simulink model "etc_demo_mix"  (R2017a)
settings: Solver=VariableStepAuto  StartTime=0.0  StopTime=1  RelTol=1e-3
values from neighbouring files (symbols this model uses):
  B = 0.0088    [sim_demo_set_para.m]
  den_p0 = R*Ks    (= 0.1305)    [sim_demo_set_para.m]
  den_p1 = L*Ks + R*B + Km*Kb    (= 0.1600195)    [sim_demo_set_para.m]
  den_p2 = L*B + R*J    (= 0.0031632)    [sim_demo_set_para.m]
  den_p3 = J*L    (= 3.15e-06)    [sim_demo_set_para.m]
  J = 0.0021    [sim_demo_set_para.m]
  K = 0.383    [sim_demo_set_para.m]
  Ks = 0.087    [sim_demo_set_para.m]
  L = 1.5e-3    (= 0.0015)    [sim_demo_set_para.m]
  num_i0 = Ks    (= 0.087)    [sim_demo_set_para.m]
  num_i1 = B    (= 0.0088)    [sim_demo_set_para.m]
  num_i2 = J    (= 0.0021)    [sim_demo_set_para.m]
  num_p0 = Km    (= 0.383)    [sim_demo_set_para.m]
  R = 1.5    [sim_demo_set_para.m]
  Tpl = 0.396    [sim_demo_set_para.m]
libraries: fl_lib x13, nesl_utility x6, simulink x1
settings Model: Creator=xiaopan-local  LastModifiedBy=xiaopan

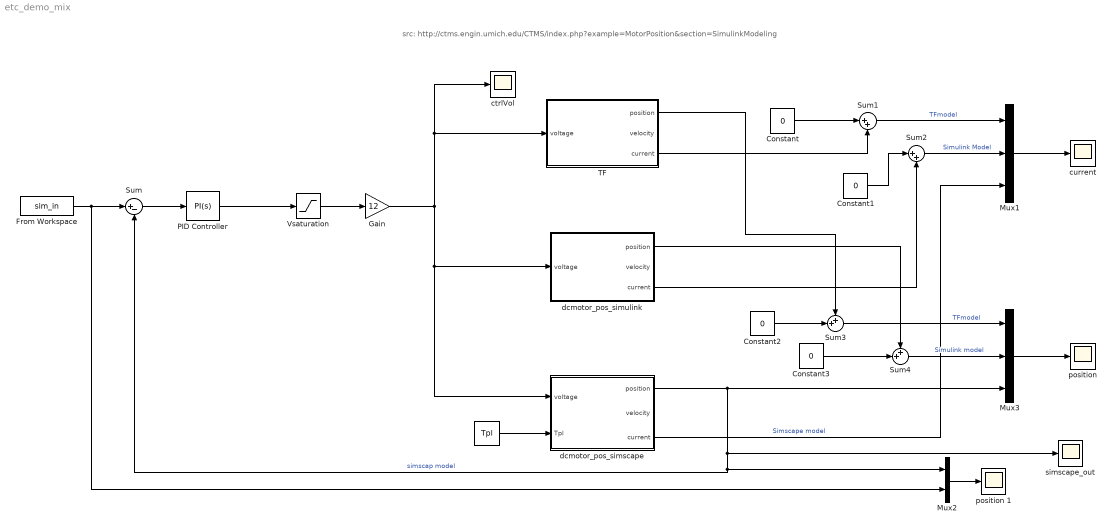
== system etc_demo_mix ==
  note: src: http://ctms.engin.umich.edu/CTMS/index.php?example=MotorPosition&section=SimulinkModeling
  " " : Constant  Value=Tpl
  Constant{,1..3} (4 alike) : Constant  Value=0
  From Workspace : FromWorkspace  VariableName=sim_in  OutDataTypeStr=double  SampleTime=0  OutputAfterFinalValue=Holding final value
  Gain : Gain  Gain=12
  Mux1 : Mux  Inputs=3
  Mux2 : Mux  Inputs=2
  Mux3 : Mux  Inputs=3
  PID Controller : simulink/Continuous/PID Controller  Controller=PI  TimeDomain=Continuous-time  SampleTime=-1  IntegratorMethod=Forward Euler  FilterMethod=Forward Euler  Form=Parallel  UseFilter=on  ControllerParametersSource=internal  P=0.76  I=0.35  D=-0.00170195605857256  N=100  InitialConditionSource=internal  InitialConditionForIntegrator=0  InitialConditionForFilter=0  ExternalReset=none  LimitOutput=off  UpperSaturationLimit=inf  LowerSaturationLimit=-inf  LinearizeAsGain=on  AntiWindupMode=none  Kb=1  TrackingMode=off  Kt=1  PParamMin=[]  PParamMax=[]  IParamMin=[]  IParamMax=[]  DParamMin=[]  DParamMax=[]  NParamMin=[]  NParamMax=[]  KbParamMin=[]  KbParamMax=[]  KtParamMin=[]  KtParamMax=[]  POutMin=[]  POutMax=[]  IOutMin=[]  IOutMax=[]  DOutMin=[]  DOutMax=[]  NOutMin=[]  NOutMax=[]  KbOutMin=[]  KbOutMax=[]  KtOutMin=[]  KtOutMax=[]  IntegratorOutMin=[]  IntegratorOutMax=[]  FilterOutMin=[]  FilterOutMax=[]  SumOutMin=[]  SumOutMax=[]  SumI1OutMin=[]  SumI1OutMax=[]  SumI2OutMin=[]  SumI2OutMax=[]  SumI3OutMin=[]  SumI3OutMax=[]  SumDOutMin=[]  SumDOutMax=[]  SaturationOutMin=[]  SaturationOutMax=[]  IntegratorContinuousStateAttributes=''  IntegratorStateMustResolveToSignalObject=off  IntegratorRTWStateStorageClass=Auto  FilterContinuousStateAttributes=''  FilterStateMustResolveToSignalObject=off  FilterRTWStateStorageClass=Auto  DifferentiatorICPrevScaledInput=0  DifferentiatorOutMin=[]  DifferentiatorOutMax=[]  InitialConditionSetting=State (most efficient)
  Sum : Sum  Inputs=|+-
  Sum1 : Sum  Inputs=|++
  Sum2 : Sum  Inputs=|++
  Sum3 : Sum  Inputs=++|
  Sum4 : Sum  Inputs=++|
  TF : Subsystem
  Vsaturation : Saturate  UpperLimit=1  LowerLimit=0
  ctrlVol : Scope
  "current " : Scope
  "dcmotor_pos_simscape " : Subsystem
  dcmotor_pos_simulink : Subsystem
  "position " : Scope
  position 1 : Scope
  simscape_out : Scope
  wires:
  Sum/1 -> PID Controller/1
  Gain/1 -> TF/1(voltage), ctrlVol/1, "dcmotor_pos_simscape "/1(voltage), dcmotor_pos_simulink/1(voltage)
  " "/1 -> "dcmotor_pos_simscape "/2(Tpl)
  Vsaturation/1 -> Gain/1
  Mux3/1 -> "position "/1
  Mux1/1 -> "current "/1
  "dcmotor_pos_simscape "/3(current) -> Mux1/3  "Simscape model"
  "dcmotor_pos_simscape "/1(position) -> Sum/2, Mux2/1, simscape_out/1, Mux3/3  "simscap model"
  TF/3(current) -> Sum1/2
  Constant/1 -> Sum1/1
  Sum1/1 -> Mux1/1  "TFmodel"
  Sum2/1 -> Mux1/2  "Simulink Model"
  Constant1/1 -> Sum2/1
  dcmotor_pos_simulink/3(current) -> Sum2/2
  TF/1("position ") -> Sum3/1
  Constant2/1 -> Sum3/2
  Sum3/1 -> Mux3/1  "TFmodel"
  Sum4/1 -> Mux3/2  "Simulink model"
  dcmotor_pos_simulink/1(position) -> Sum4/1
  Constant3/1 -> Sum4/2
  From Workspace/1 -> Mux2/2, Sum/1
  Mux2/1 -> position 1/1
  PID Controller/1 -> Vsaturation/1

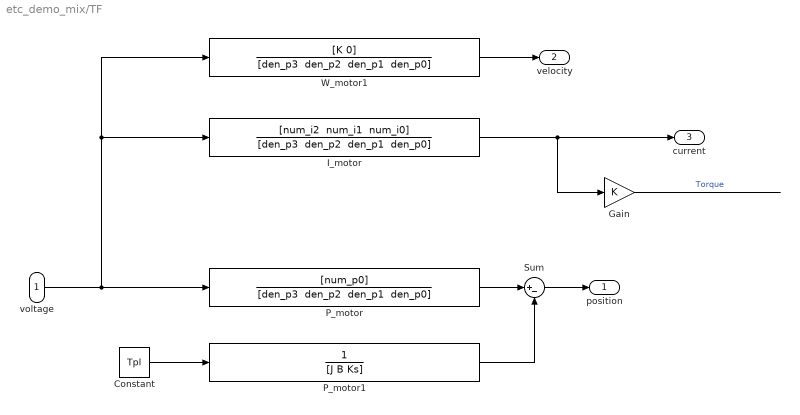
== system etc_demo_mix/TF ==
  voltage : Inport
  Constant : Constant  Value=Tpl
  Gain : Gain  Gain=K
  I_motor : TransferFcn  Numerator="[num_i2  num_i1  num_i0]"  Denominator="[den_p3  den_p2  den_p1  den_p0]"
  P_motor : TransferFcn  Numerator=[num_p0]  Denominator="[den_p3  den_p2  den_p1  den_p0]"
  P_motor1 : TransferFcn  Denominator=[J B Ks]
  Sum : Sum  Inputs=|+-
  W_motor1 : TransferFcn  Numerator=[K 0]  Denominator="[den_p3  den_p2  den_p1  den_p0]"
  "position " : Outport
  velocity : Outport  Port=2
  current : Outport  Port=3
  wires:
  voltage/1 -> I_motor/1, W_motor1/1, P_motor/1
  W_motor1/1 -> velocity/1
  I_motor/1 -> Gain/1, current/1
  Constant/1 -> P_motor1/1
  P_motor/1 -> Sum/1
  P_motor1/1 -> Sum/2
  Sum/1 -> "position "/1
  Gain/1 -> ?  "Torque"

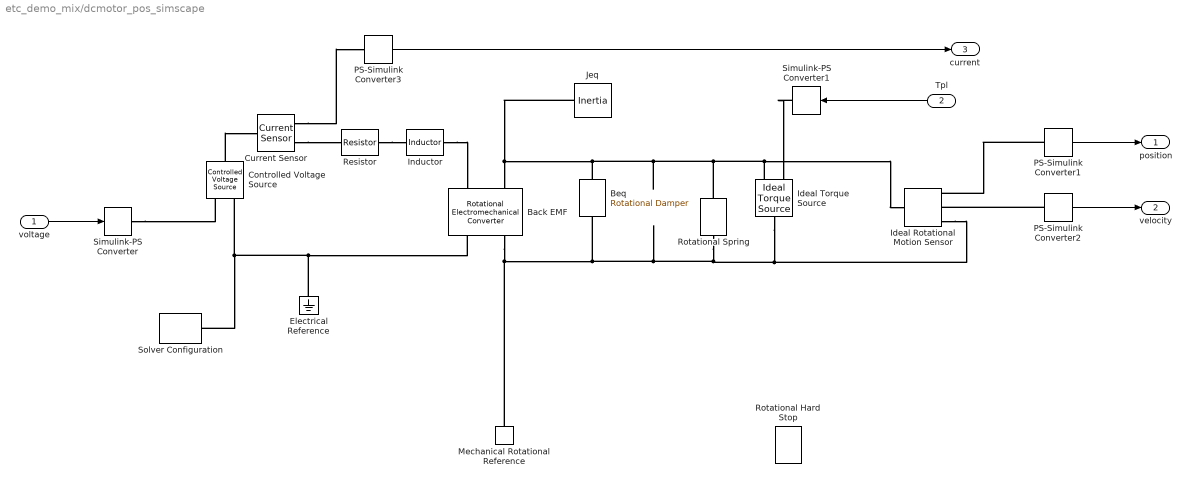
== system etc_demo_mix/dcmotor_pos_simscape  ==
  voltage : Inport
  Tpl : Inport  Port=2
  Back EMF : fl_lib/Electrical/Electrical Elements/Rotational Electromechanical Converter  K=K V/(rad/s)  i_specify=off  i_priority=None  i=0 A  i_nominal_specify=off  i_nominal_unit=A  i_nominal_value=1  v_specify=off  v_priority=None  v=0 V  v_nominal_specify=off  v_nominal_unit=V  v_nominal_value=1  t_specify=off  t_priority=None  t=0 N*m  t_nominal_specify=off  t_nominal_unit=N*m  t_nominal_value=1  w_specify=off  w_priority=None  w=0 rad/s  w_nominal_specify=off  w_nominal_unit=rad/s  w_nominal_value=1
      settings: SourceProductName=Simscape
  Beq : fl_lib/Mechanical/Rotational Elements/Rotational Damper  D=B N*m/(rad/s)  w_specify=off  w_priority=None  w=0 rad/s  w_nominal_specify=off  w_nominal_unit=rad/s  w_nominal_value=1  t_specify=off  t_priority=None  t=0 N*m  t_nominal_specify=off  t_nominal_unit=N*m  t_nominal_value=1
  Controlled Voltage Source : fl_lib/Electrical/Electrical Sources/Controlled Voltage Source
  Current Sensor : fl_lib/Electrical/Electrical Sensors/Current Sensor
  Electrical Reference : fl_lib/Electrical/Electrical Elements/Electrical Reference
  Ideal Rotational Motion Sensor : fl_lib/Mechanical/Mechanical Sensors/Ideal Rotational Motion Sensor  offset=0 rad
  Ideal Torque Source : fl_lib/Mechanical/Mechanical Sources/Ideal Torque Source
  Inductor : fl_lib/Electrical/Electrical Elements/Inductor  l=L mH  r=0 Ohm  g=0 1/Ohm  i_specify=off  i_priority=None  i=0 A  i_nominal_specify=off  i_nominal_unit=A  i_nominal_value=1  v_specify=off  v_priority=None  v=0 V  v_nominal_specify=off  v_nominal_unit=V  v_nominal_value=1  i_L_specify=off  i_L_priority=High  i_L=0 A  i_L_nominal_specify=off  i_L_nominal_unit=A  i_L_nominal_value=1
  Jeq : fl_lib/Mechanical/Rotational Elements/Inertia  inertia=J kg*m^2  w_specify=off  w_priority=High  w=0 rad/s  w_nominal_specify=off  w_nominal_unit=rad/s  w_nominal_value=1  t_specify=off  t_priority=None  t=0 N*m  t_nominal_specify=off  t_nominal_unit=N*m  t_nominal_value=1
      settings: LogSimulationData=on
  Mechanical Rotational Reference : fl_lib/Mechanical/Rotational Elements/Mechanical Rotational Reference
  PS-Simulink Converter1 : nesl_utility/PS-Simulink Converter  PhysicalDomain=network_engine_domain  SubClassName=ps_output  LeftPortType=input  RightPortType=output  PseudoPeriodic=off  Frequencies=[]  Unit=1  AffineConversion=off
  PS-Simulink Converter2 : nesl_utility/PS-Simulink Converter  PhysicalDomain=network_engine_domain  SubClassName=ps_output  LeftPortType=input  RightPortType=output  PseudoPeriodic=off  Frequencies=[]  Unit=1  AffineConversion=off
  PS-Simulink Converter3 : nesl_utility/PS-Simulink Converter  PhysicalDomain=network_engine_domain  SubClassName=ps_output  LeftPortType=input  RightPortType=output  PseudoPeriodic=off  Frequencies=[]  Unit=1  AffineConversion=off
  Resistor : fl_lib/Electrical/Electrical Elements/Resistor  R=R Ohm  i_specify=off  i_priority=None  i=0 A  i_nominal_specify=off  i_nominal_unit=A  i_nominal_value=1  v_specify=off  v_priority=None  v=0 V  v_nominal_specify=off  v_nominal_unit=V  v_nominal_value=1
  Rotational Hard Stop : fl_lib/Mechanical/Rotational Elements/Rotational Hard Stop  upper_bnd=180 deg  lower_bnd=0 rad  stiff_up=1e6 N*m/rad  stiff_low=1e6 N*m/rad  D_up=0.01 N*m/(rad/s)  D_low=0.01 N*m/(rad/s)  w_specify=off  w_priority=None  w=0 rad/s  w_nominal_specify=off  w_nominal_unit=rad/s  w_nominal_value=1  t_specify=off  t_priority=None  t=0 N*m  t_nominal_specify=off  t_nominal_unit=N*m  t_nominal_value=1  phi_specify=off  phi_priority=High  phi=0 rad  phi_nominal_specify=off  phi_nominal_unit=rad  phi_nominal_value=1
      settings: SourceProductName=Simscape  SourceProductBaseCode=SS
  Rotational Spring : fl_lib/Mechanical/Rotational Elements/Rotational Spring  spr_rate=Ks N*m/rad  w_specify=off  w_priority=None  w=0 rad/s  w_nominal_specify=off  w_nominal_unit=rad/s  w_nominal_value=1  t_specify=off  t_priority=None  t=0 N*m  t_nominal_specify=off  t_nominal_unit=N*m  t_nominal_value=1  phi_specify=off  phi_priority=High  phi=0 rad  phi_nominal_specify=off  phi_nominal_unit=rad  phi_nominal_value=1
      settings: SourceProductName=Simscape
  Simulink-PS Converter : nesl_utility/Simulink-PS Converter  PhysicalDomain=network_engine_domain  SubClassName=ps_input  LeftPortType=input  RightPortType=output  PseudoPeriodic=off  Frequencies=[]  NoiseDistribution=none  NoiseParameters=[]  Unit=1  AffineConversion=off  FilteringAndDerivatives=provide  SimscapeFilterOrder=1  InputFilterTimeConstant=0.001  UdotUserProvided=0
  Simulink-PS Converter1 : nesl_utility/Simulink-PS Converter  PhysicalDomain=network_engine_domain  SubClassName=ps_input  LeftPortType=input  RightPortType=output  PseudoPeriodic=off  Frequencies=[]  NoiseDistribution=none  NoiseParameters=[]  Unit=1  AffineConversion=off  FilteringAndDerivatives=provide  SimscapeFilterOrder=1  InputFilterTimeConstant=0.001  UdotUserProvided=0
  Solver Configuration : nesl_utility/Solver Configuration  PhysicalDomain=network_engine_domain  SubClassName=solver  LeftPortType=input  RightPortType=generic  Accelerate=off  Tones=[]  Harmonics=[]  SimulateNoise=off  Profile=off  UseLocalSampling=off  EnableSwitchedLinearOptims=on  FrequencyDomain=off  UseCCode=off  RelTol=0.001  AbsTol=1e-06  MinStep=1e-09  ToWorkspace=off  RevertToSquareIcSolve=off  NumHomotopyIterations=100  PhasorMode=off  PhasorModeNumHarmonics=1  OverrideAbsTol=off  DoDC=off  ResidualTolerance=1e-09  UseLocalSolver=off  LocalSolverChoice=NE_BACKWARD_EULER_ADVANCER  LocalSolverSampleTime=0.001  DoFixedCost=off  MaxNonlinIter=3  MaxModeIter=2  LinearAlgebra=Sparse  DelaysMemoryBudget=1024  AutomaticFiltering=on  FilteringTimeConstant=0.001
  position : Outport
  velocity : Outport  Port=2
  current : Outport  Port=3
  wires:
  PS-Simulink Converter2/1 -> velocity/1
  PS-Simulink Converter1/1 -> position/1
  voltage/1 -> Simulink-PS Converter/1
  PS-Simulink Converter3/1 -> current/1
  Tpl/1 -> Simulink-PS Converter1/1
  connections:
  Resistor/RConn1 -- Inductor/LConn1
  Inductor/RConn1 -- Back EMF/LConn1
  Mechanical Rotational Reference/LConn1 -- Back EMF/RConn2 -- Beq/RConn1 -- Rotational Spring/LConn1 -- Ideal Rotational Motion Sensor/RConn1 -- Ideal Torque Source/LConn1
  Electrical Reference/LConn1 -- Back EMF/RConn1 -- Solver Configuration/RConn1 -- Controlled Voltage Source/RConn2
  PS-Simulink Converter1/LConn1 -- Ideal Rotational Motion Sensor/RConn3
  PS-Simulink Converter2/LConn1 -- Ideal Rotational Motion Sensor/RConn2
  Current Sensor/RConn2 -- Resistor/LConn1
  Current Sensor/RConn1 -- PS-Simulink Converter3/LConn1
  Controlled Voltage Source/LConn1 -- Current Sensor/LConn1
  Simulink-PS Converter/RConn1 -- Controlled Voltage Source/RConn1
  Simulink-PS Converter1/RConn1 -- Ideal Torque Source/RConn1
  Jeq/LConn1 -- Back EMF/LConn2 -- Beq/LConn1 -- Ideal Torque Source/RConn2 -- Ideal Rotational Motion Sensor/LConn1 -- Rotational Spring/RConn1

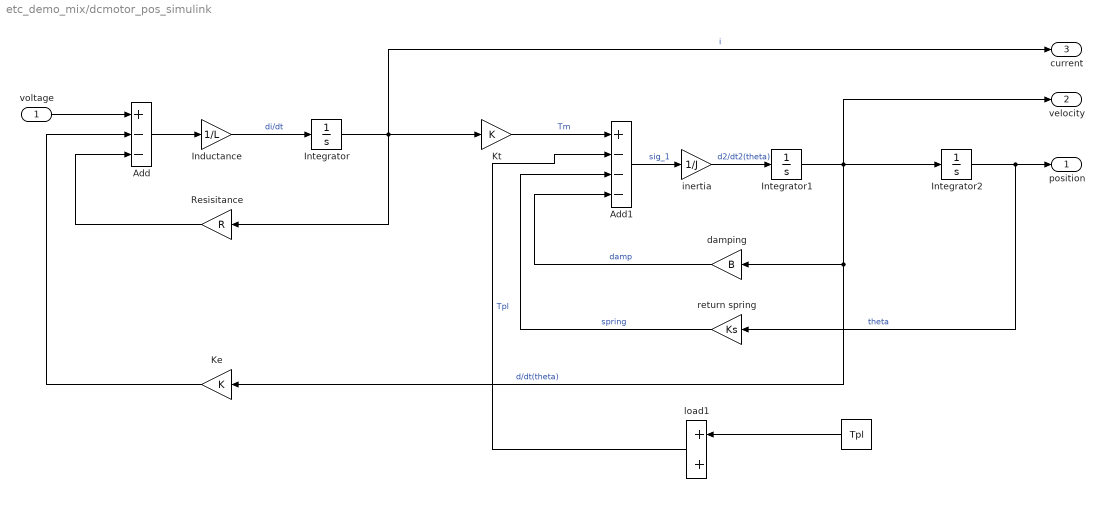
== system etc_demo_mix/dcmotor_pos_simulink ==
  voltage : Inport
  " " : Constant  Value=Tpl
  Add : Sum  Inputs=+--
  Add1 : Sum  Inputs=+---
  "Inductance " : Gain  Gain=1/L
  Integrator : Integrator
  Integrator1 : Integrator
  Integrator2 : Integrator
  Ke : Gain  Gain=K
  Kt : Gain  Gain=K
  Resisitance : Gain  Gain=R
  damping : Gain  Gain=B
  inertia : Gain  Gain=1/J
  load1 : Sum
  return spring : Gain  Gain=Ks
  position : Outport
  velocity : Outport  Port=2
  current : Outport  Port=3
  wires:
  voltage/1 -> Add/1
  Add/1 -> "Inductance "/1
  Add1/1 -> inertia/1  "sig_1"
  "Inductance "/1 -> Integrator/1  "di/dt"
  inertia/1 -> Integrator1/1  "d2/dt2(theta)"
  Integrator2/1 -> return spring/1, position/1  "theta"
  Resisitance/1 -> Add/3
  damping/1 -> Add1/4  "damp"
  Integrator1/1 -> Integrator2/1, velocity/1, Ke/1, damping/1  "d/dt(theta)"
  Ke/1 -> Add/2
  Kt/1 -> Add1/1  "Tm"
  Integrator/1 -> current/1, Kt/1, Resisitance/1  "i"
  " "/1 -> load1/1
  load1/1 -> Add1/2  "Tpl"
  return spring/1 -> Add1/3  "spring"
